simulink model "P_PI_4opamp_blocks"  (R2019b)
settings: Solver=VariableStepAuto  StartTime=0.0  StopTime=15  RelTol=1e-3
settings Model: Creator=robom  LastModifiedBy=robom
settings DataIOCC: SaveOutput=off  ReturnWorkspaceOutputs=off
settings SFSimCC: CustomCodeUndefinedFunction=UseInterfaceOnly

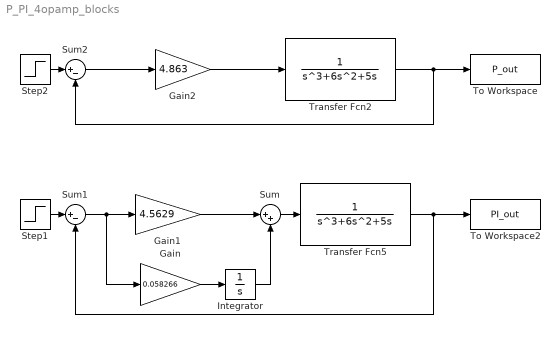
== system P_PI_4opamp_blocks ==
  Gain : Gain  Gain=0.058266
  Gain1 : Gain  Gain=4.5629
  Gain2 : Gain  Gain=4.863
  Integrator : Integrator
  Step1 : Step  Time=0  SampleTime=0
  Step2 : Step  Time=0  SampleTime=0
  Sum : Sum  Inputs=|++
  Sum1 : Sum  Inputs=|+-
  Sum2 : Sum  Inputs=|+-
  To Workspace : ToWorkspace  VariableName=P_out  SampleTime=-1
      settings: Save2DSignal=2-D array (concatenate along first dimension)
  To Workspace2 : ToWorkspace  VariableName=PI_out  SampleTime=-1
      settings: Save2DSignal=2-D array (concatenate along first dimension)
  Transfer Fcn2 : TransferFcn  Denominator=[1 6 5 0]
  Transfer Fcn5 : TransferFcn  Denominator=[1 6 5 0]
  wires:
  Step2/1 -> Sum2/1
  Transfer Fcn2/1 -> To Workspace/1, Sum2/2
  Gain2/1 -> Transfer Fcn2/1
  Sum2/1 -> Gain2/1
  Sum1/1 -> Gain/1, Gain1/1
  Transfer Fcn5/1 -> To Workspace2/1, Sum1/2
  Step1/1 -> Sum1/1
  Gain1/1 -> Sum/1
  Sum/1 -> Transfer Fcn5/1
  Gain/1 -> Integrator/1
  Integrator/1 -> Sum/2
